simulink library "Driveshaft_ShaftsAll"  (R2026a)
settings: Solver=VariableStepAuto
undefined symbols (not defined in the file): Axle1D, AxleIn, Driveshaft, Housing, Right, Shaft, Shaft1D, Shaft3D, Vehicle, Visual, X, Y, Z
libraries: sm_lib x27, $bdroot x6, fl_lib x4, nesl_utility x2, sm_car_lib x2, Differential_Components x1
Description:
  | Component of Simscape Vehicle Templates Library
  | 
  | Copyright 2018-2026 The MathWorks, Inc.
settings Model: Creator=smiller  LastModifiedBy=smiller

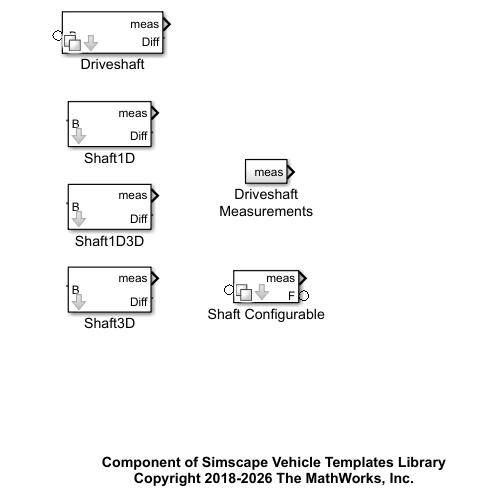
[thumbnail: Simulink's stored preview of the top-level diagram]
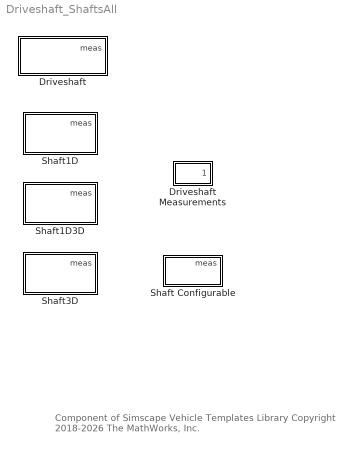
== system Driveshaft_ShaftsAll ==
  note: Component of Simscape Vehicle Templates Library
      | Copyright 2018-2026 The MathWorks, Inc.
  Driveshaft : Subsystem  Variant=on  VariantControl=Variant1  mask(Driveshaft Assembly){popup_leftRight=Right, Driveshaft=Vehicle.Powertrain.Driveline.DriveshaftFR, VariantLabel=Vehicle.Powertrain.Driveline.DriveshaftFR.class.Value, InitTriggerDropdown=1}
      mask prompts: popup_leftRight "Left/Right"; Driveshaft "Driveshaft Parameters"; VariantLabel "Variant Label"; InitTriggerDropdown "Initialization Trigger Dropdown"
      mask help: Models driveshaft and connections to differential and wheels. Joints can be configured to permit plunge at inner or outer joints.
      mask init:
      | curblk = gcb;
      | 
      | % Find other left/right blocks
      | h = sm_car_lib_find_leftright_blocks(curblk);
      | 
      | % Set left/right
      | for i=1:length(h)
      |     try % Avoid setting parameter within library links
      |         set_param(h(i),'popup_leftRight',get_param(curblk,'popup_leftRight'));
      |     end
      | end
      | 
      | % Set variant for this block 
      | set_param(curblk,'LabelModeActiveChoice',VariantLabel);
      | 
      | % Trigger Mask Initialization for 
      | % variant subsystems below this level
      | sm_car_lib_maskInitTrigger(curblk)
      settings: AttributesFormatString=%<ActiveVariant>
      mask TypeOptions popup_leftRight: Left | Right
      mask TypeOptions InitTriggerDropdown: 0 | 1
      mask Display: disp(' ');
  Driveshaft Measurements : Subsystem
  Shaft Configurable : Subsystem  Variant=on  VariantControl=Variant1  mask(Shaft (Configurable)){popup_leftRight=Right, Shaft=Vehicle.Powertrain.Driveline.DriveshaftFL.Shaft, VariantLabel=Vehicle.Powertrain.Driveline.DriveshaftFL.Shaft.class.Value, InitTriggerDropdown=1, clr_shaft=Visual.Driveshaft.clr, opc_shaft=Visual.part.opc, rad_shaft=Visual.Driveshaft.rad}
      mask prompts: popup_leftRight "Left/Right"; Shaft "Shaft Parameters"; VariantLabel "Variant Label"; InitTriggerDropdown "Initialization Trigger Dropdown"; clr_shaft "Color [RGB]"; opc_shaft "Opacity (0-1)"; rad_shaft "Radius (m)"
      mask help: Models a shaft (rigid or flexible).
      mask init:
      | curblk = gcb;
      | 
      | % Find other left/right blocks
      | h = sm_car_lib_find_leftright_blocks(curblk);
      | 
      | % Set left/right
      | for i=1:length(h)
      |     try % Avoid setting parameter within library links
      |         set_param(h(i),'popup_leftRight',get_param(curblk,'popup_leftRight'));
      |     end
      | end
      | 
      | % Set variant for this block 
      | set_param(curblk,'LabelModeActiveChoice',VariantLabel);
      | 
      | % Trigger Mask Initialization for 
      | % variant subsystems below this level
      | sm_car_lib_maskInitTrigger(curblk)
      mask TypeOptions popup_leftRight: Left | Right
      mask TypeOptions InitTriggerDropdown: 0 | 1
      mask DialogControl cont_vis_shaft Prompt: Visualization
      mask Display: disp(' ')
  Shaft1D : Subsystem  VariantControl=Shaft1D  mask(Driveshaft Assembly (1D)){}
      mask help: Models a shaft as a 1D mechanical connection.
  Shaft1D3D : Subsystem  VariantControl=Shaft1D3D  mask(Driveshaft Assembly (1D and 3D)){popup_leftRight=Right, drv_sha_drvsh_m=Driveshaft.Shaft.m.Value, clr_drv_sha_hp=Visual.hp.clr, opc_drv_sha_hp=Visual.hp.opc, rad_drv_sha_hp=Visual.hp.rad, clr_drv_sha_jnt=Visual.DriveshaftCVs.clr, opc_drv_sha_jnt=Visual.part.opc, rad_drv_sha_jnt=Visual.DriveshaftCVs.rad, clr_drv_sha_drvsh=Visual.Driveshaft.clr, opc_drv_sha_drvsh=Visual.part.opc, rad_drv_sha_drvsh=Visual.Driveshaft.rad, len_drv_sha_drvsh=Driveshaft.Shaft.l.Value}
      mask prompts: popup_leftRight "Left/Right"; drv_sha_drvsh_m "Driveshaft Mass (kg)"; len_drv_sha_drvsh "Driveshaft Length (m)"
      mask help: Models a shaft with a 1D mechanical connection for transmitting power and a non-rotating 3D connection for inertia and visualization.
      mask TypeOptions popup_leftRight: AxleInboard/popup_leftRight | Shaft/popup_leftRight | Transaxle/popup_leftRight
      mask TypeOptions drv_sha_drvsh_m: Shaft/shaft_m
      mask TypeOptions clr_drv_sha_hp:
      | Vis HP
      | Transaxle/GraphicDiffuseColor
      mask TypeOptions opc_drv_sha_hp:
      | Vis HP
      | Transaxle/GraphicOpacity
      mask TypeOptions rad_drv_sha_hp:
      | Vis HP
      | Transaxle/SphereRadius
      mask TypeOptions clr_drv_sha_jnt:
      | Vis CV Joint
      | Inboard/GraphicDiffuseColor | Vis CV Joint
      | Outboard/GraphicDiffuseColor
      mask TypeOptions opc_drv_sha_jnt:
      | Vis CV Joint
      | Inboard/GraphicOpacity | Vis CV Joint
      | Outboard/GraphicOpacity
      mask TypeOptions rad_drv_sha_jnt:
      | Vis CV Joint
      | Inboard/SphereRadius | Vis CV Joint
      | Outboard/SphereRadius
      mask TypeOptions clr_drv_sha_drvsh: Shaft/clr_shaft
      mask TypeOptions opc_drv_sha_drvsh: Shaft/opc_shaft
      mask TypeOptions rad_drv_sha_drvsh: Shaft/rad_shaft
      mask TypeOptions len_drv_sha_drvsh: Shaft/len_shaft
      mask DialogControl cont_vis_drv_sha Prompt: Visualization
      mask DialogControl text_vis_drv_sha_clr Prompt: Color [RGB]
      mask DialogControl text_vis_drv_sha_opc Prompt: Opac. (0-1)
      mask DialogControl text_vis_drv_sha_rad Prompt: Radius (m)
      mask DialogControl text_vis_drv_sha_hp Prompt: Hardpoints
      mask DialogControl text_vis_drv_sha_joints Prompt: Joints
      mask DialogControl text_vis_drv_sha_drvsh Prompt: Driveshaft
  Shaft3D : Subsystem  VariantControl=Shaft3D  mask(Driveshaft Assembly (3D)){popup_leftRight=Right, Driveshaft=Driveshaft, InitTriggerDropdown=1, clr_drv_sha_hp=Visual.hp.clr, opc_drv_sha_hp=Visual.hp.opc, rad_drv_sha_hp=Visual.hp.rad, clr_drv_sha_jnt=Visual.DriveshaftCVs.clr, opc_drv_sha_jnt=Visual.part.opc, rad_drv_sha_jnt=Visual.DriveshaftCVs.rad, clr_drv_sha_drvsh=Visual.Driveshaft.clr, opc_drv_sha_drvsh=Visual.part.opc, rad_drv_sha_drvsh=Visual.Driveshaft.rad}
      mask prompts: popup_leftRight "Left/Right"; Driveshaft "Driveshaft Parameters"; InitTriggerDropdown "Initialization Trigger Dropdown"
      mask help: Models a driveshaft assembly with CV joints and a shaft. The joints can be configured to permit plunge at the inboard or outboard joint. The shaft can be rigid or flexible.
      mask init:
      | curblk = gcb;
      | 
      | % Trigger Mask Initialization for 
      | % variant subsystems below this level
      | sm_car_lib_maskInitTrigger(curblk)
      mask TypeOptions popup_leftRight: AxleInboard/popup_leftRight | Shaft/popup_leftRight
      mask TypeOptions InitTriggerDropdown: 0 | 1
      mask TypeOptions clr_drv_sha_hp:
      | Vis HP
      | Transaxle/GraphicDiffuseColor
      mask TypeOptions opc_drv_sha_hp:
      | Vis HP
      | Transaxle/GraphicOpacity
      mask TypeOptions rad_drv_sha_hp:
      | Vis HP
      | Transaxle/SphereRadius
      mask TypeOptions clr_drv_sha_jnt:
      | Vis CV Joint
      | Inboard/GraphicDiffuseColor | Vis CV Joint
      | Outboard/GraphicDiffuseColor
      mask TypeOptions opc_drv_sha_jnt:
      | Vis CV Joint
      | Inboard/GraphicOpacity | Vis CV Joint
      | Outboard/GraphicOpacity
      mask TypeOptions rad_drv_sha_jnt:
      | Vis CV Joint
      | Inboard/SphereRadius | Vis CV Joint
      | Outboard/SphereRadius
      mask TypeOptions clr_drv_sha_drvsh: Shaft/clr_shaft
      mask TypeOptions opc_drv_sha_drvsh: Shaft/opc_shaft
      mask TypeOptions rad_drv_sha_drvsh: Shaft/rad_shaft
      mask DialogControl cont_vis_drv_sha Prompt: Visualization
      mask DialogControl text_vis_drv_sha_clr Prompt: Color [RGB]
      mask DialogControl text_vis_drv_sha_opc Prompt: Opac. (0-1)
      mask DialogControl text_vis_drv_sha_rad Prompt: Radius (m)
      mask DialogControl text_vis_drv_sha_hp Prompt: Hardpoints
      mask DialogControl text_vis_drv_sha_joints Prompt: Joints
      mask DialogControl text_vis_drv_sha_drvsh Prompt: Driveshaft

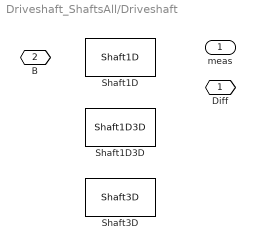
== system Driveshaft_ShaftsAll/Driveshaft ==
  Shaft1D : $bdroot/Shaft1D  VariantControl=Shaft1D
  Shaft1D3D : $bdroot/Shaft1D3D  VariantControl=Shaft1D3D  popup_leftRight=Right  drv_sha_drvsh_m=Driveshaft.Shaft.m.Value  clr_drv_sha_hp=Visual.hp.clr  opc_drv_sha_hp=Visual.hp.opc  rad_drv_sha_hp=Visual.hp.rad  clr_drv_sha_jnt=Visual.DriveshaftCVs.clr  opc_drv_sha_jnt=Visual.part.opc  rad_drv_sha_jnt=Visual.DriveshaftCVs.rad  clr_drv_sha_drvsh=Visual.Driveshaft.clr  opc_drv_sha_drvsh=Visual.part.opc  rad_drv_sha_drvsh=Visual.Driveshaft.rad  len_drv_sha_drvsh=Driveshaft.Shaft.l.Value
  Shaft3D : $bdroot/Shaft3D  VariantControl=Shaft3D  popup_leftRight=Right  Driveshaft=Driveshaft  InitTriggerDropdown=1  clr_drv_sha_hp=Visual.hp.clr  opc_drv_sha_hp=Visual.hp.opc  rad_drv_sha_hp=Visual.hp.rad  clr_drv_sha_jnt=Visual.DriveshaftCVs.clr  opc_drv_sha_jnt=Visual.part.opc  rad_drv_sha_jnt=Visual.DriveshaftCVs.rad  clr_drv_sha_drvsh=Visual.Driveshaft.clr  opc_drv_sha_drvsh=Visual.part.opc  rad_drv_sha_drvsh=Visual.Driveshaft.rad
  Diff : PMIOPort  Side=Right
  " B" : PMIOPort  Port=2  Side=Left
  meas : Outport  VectorParamsAs1DForOutWhenUnconnected=off

== system Driveshaft_ShaftsAll/Driveshaft Measurements ==
  Bus Creator : BusCreator  Inputs=2
  Zero : Constant  Value=0  OutDataTypeStr=Inherit: Inherit via back propagation
  Zero1 : Constant  Value=0  OutDataTypeStr=Inherit: Inherit via back propagation
  meas : Outport  VectorParamsAs1DForOutWhenUnconnected=off
  wires:
  Bus Creator/1 -> meas/1
  Zero1/1 -> Bus Creator/2  "q"
  Zero/1 -> Bus Creator/1  "w"

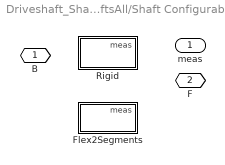
== system Driveshaft_ShaftsAll/Shaft Configurable ==
  Flex2Segments : Subsystem  VariantControl=Flex2Segments  mask{popup_leftRight=Right, shaft_m=Shaft.m.Value, len_shaft=Shaft.l.Value, shaft_K=Shaft.K.Value, shaft_d=Shaft.d.Value, clr_shaft=clr_shaft, opc_shaft=opc_shaft, rad_shaft=rad_shaft}
      mask prompts: popup_leftRight "Left/Right"; shaft_m "Shaft Mass (kg)"; len_shaft "Shaft Length (m)"; shaft_K "Shaft Stiffness (N*m/rad)"; shaft_d "Shaft Damping (N*m/(rad/s))"; clr_shaft "Color [RGB]"; opc_shaft "Opacity (0-1)"; rad_shaft "Radius (m)"
      mask init:
      | if(popup_leftRight == 1)
      |     rhs_shaft = 1;
      | elseif(popup_leftRight == 2)
      |     rhs_shaft = -1;
      | end
      mask TypeOptions popup_leftRight: Left | Right
      mask TypeOptions shaft_m: Shaft/Mass
      mask TypeOptions shaft_K:
      | Revolute
      | Flex/SpringStiffness
      mask TypeOptions shaft_d:
      | Revolute
      | Flex/DampingCoefficient
      mask TypeOptions clr_shaft: Shaft/GraphicDiffuseColor
      mask TypeOptions opc_shaft: Shaft/GraphicOpacity
      mask TypeOptions rad_shaft: Shaft/CylinderRadius
      mask DialogControl cont_vis_shaft Prompt: Visualization
  Rigid : Subsystem  VariantControl=Rigid  mask{popup_leftRight=Right, shaft_m=Shaft.m.Value, len_shaft=Shaft.l.Value, clr_shaft=clr_shaft, opc_shaft=opc_shaft, rad_shaft=rad_shaft}
      mask prompts: popup_leftRight "Left/Right"; shaft_m "Shaft Mass (kg)"; len_shaft "Shaft Length (m)"; clr_shaft "Color [RGB]"; opc_shaft "Opacity (0-1)"; rad_shaft "Radius (m)"
      mask init:
      | if(popup_leftRight == 1)
      |     rhs_shaft = 1;
      | elseif(popup_leftRight == 2)
      |     rhs_shaft = -1;
      | end
      mask TypeOptions popup_leftRight: Left | Right
      mask TypeOptions shaft_m: Shaft/Mass
      mask TypeOptions clr_shaft: Shaft/GraphicDiffuseColor
      mask TypeOptions opc_shaft: Shaft/GraphicOpacity
      mask TypeOptions rad_shaft: Shaft/CylinderRadius
      mask DialogControl cont_vis_shaft Prompt: Visualization
  " B" : PMIOPort  Side=Left
  " F" : PMIOPort  Port=2  Side=Right
  " meas" : Outport  VectorParamsAs1DForOutWhenUnconnected=off

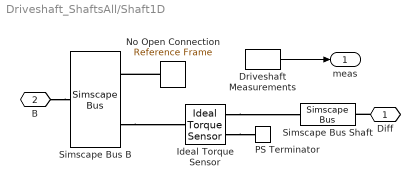
== system Driveshaft_ShaftsAll/Shaft1D ==
  Driveshaft Measurements : $bdroot/Driveshaft Measurements  SystemSampleTime=-1  VariantActivationTime=update diagram  EmptyChoice=off  PassThrough=off  PassThroughVariantControl=(default)  EmptyChoiceVariantControl=(default)  AllowFlexibleInterface=on  Latency=0  AutoFrameSizeCalculation=off
  Ideal Torque Sensor : fl_lib/Mechanical/Mechanical Sensors/Ideal Torque Sensor
  No Open Connection : sm_lib/Frames and Transforms/Reference Frame
  PS Terminator : fl_lib/Physical Signals/Sinks/PS Terminator
  Simscape Bus B : SimscapeBus  HierarchyStrings=AxleIn;Axle1D
  Simscape Bus Shaft : SimscapeBus  HierarchyStrings=Shaft1D
  Diff : PMIOPort  Side=Right
  B : PMIOPort  Port=2  Side=Left
  meas : Outport  VectorParamsAs1DForOutWhenUnconnected=off
  wires:
  Driveshaft Measurements/1 -> meas/1
  connections:
  No Open Connection/RConn1 -- Simscape Bus B/LConn1
  B/RConn1 -- Simscape Bus B/RConn1
  Ideal Torque Sensor/RConn2 -- PS Terminator/LConn1
  Diff/RConn1 -- Simscape Bus Shaft/RConn1
  Ideal Torque Sensor/RConn1 -- Simscape Bus Shaft/LConn1
  Simscape Bus B/LConn2 -- Ideal Torque Sensor/LConn1

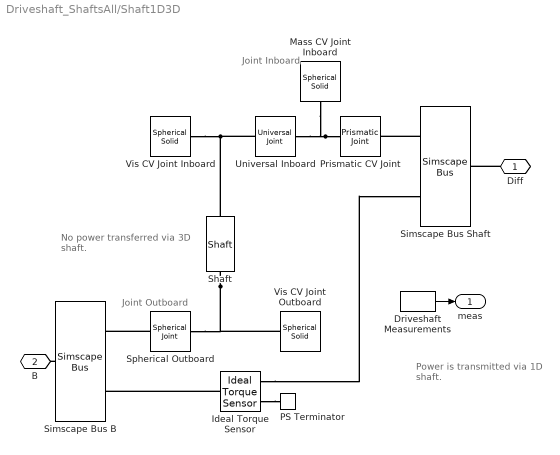
== system Driveshaft_ShaftsAll/Shaft1D3D ==
  note: Joint Inboard
  note: Joint Outboard
  note: No power transferred
      | via 3D shaft.
  note: Power is transmitted via 1D shaft.
  Driveshaft Measurements : $bdroot/Driveshaft Measurements  SystemSampleTime=-1  VariantActivationTime=update diagram  EmptyChoice=off  PassThrough=off  PassThroughVariantControl=(default)  EmptyChoiceVariantControl=(default)  AllowFlexibleInterface=on  Latency=0  AutoFrameSizeCalculation=off
  Ideal Torque Sensor : fl_lib/Mechanical/Mechanical Sensors/Ideal Torque Sensor
  Mass CV Joint Inboard : sm_lib/Body Elements/Spherical Solid  SphereRadius=5e-3  SphereRadiusUnits=m  ExportEntireGeometry=off  InertiaType=CalculateFromGeometry  BasedOnType=Density  Density=1000  DensityUnits=kg/m^3  Mass=1  MassUnits=kg  CenterOfMass=[0 0 0]  CenterOfMassUnits=m  MomentsOfInertia=[1 1 1]  MomentsOfInertiaUnits=kg*m^2  ProductsOfInertia=[0 0 0]  ProductsOfInertiaUnits=kg*m^2  GraphicType=FromGeometry  MarkerShape=Sphere  MarkerSize=10  GraphicVisPropType=SimpleVisualProperties  GraphicDiffuseColor=[0.5 0.5 0.5]  GraphicOpacity=1  GraphicSpecularColor=[0.5 0.5 0.5 1.0]  GraphicAmbientColor=[0.15 0.15 0.15 1.0]  GraphicEmissiveColor=[0.0 0.0 0.0 1.0]  GraphicShininess=75  DoExposeReferenceFrame=on  SerializedFrames=<Frames/>
  PS Terminator : fl_lib/Physical Signals/Sinks/PS Terminator
  Prismatic CV Joint : sm_lib/Joints/Prismatic Joint  JointMode=Normal  CompositeWrenchDir=FollowerOnBase  CompositeWrenchFrame=BaseFrame  SenseConstraintForce=off  SenseConstraintTorque=off  SenseTotalForce=off  SenseTotalTorque=off  PositionTargetSpecify=off  PositionTargetPriority=High  PositionTargetValue=0  PositionTargetValueUnits=m  VelocityTargetSpecify=off  VelocityTargetPriority=High  VelocityTargetValue=0  VelocityTargetValueUnits=m/s  EquilibriumPosition=0  EquilibriumPositionUnits=m  SpringStiffness=0  SpringStiffnessUnits=N/m  DampingCoefficient=0  DampingCoefficientUnits=N/(m/s)  LowerLimitSpecify=off  LowerLimitBound=-1  LowerLimitBoundUnits=m  LowerLimitStiffness=1e6  LowerLimitStiffnessUnits=N/m  LowerLimitDamping=1e3  LowerLimitDampingUnits=N/(m/s)  LowerLimitTransitionRegionWidth=1e-4  LowerLimitTransitionRegionWidthUnits=m  UpperLimitSpecify=off  UpperLimitBound=1  UpperLimitBoundUnits=m  UpperLimitStiffness=1e6  UpperLimitStiffnessUnits=N/m  UpperLimitDamping=1e3  UpperLimitDampingUnits=N/(m/s)  UpperLimitTransitionRegionWidth=1e-4  UpperLimitTransitionRegionWidthUnits=m  TorqueActuationMode=NoTorque  MotionActuationMode=ComputedMotion  SensePosition=off  SenseVelocity=off  SenseAcceleration=off  SenseTorqueForce=off  SenseLowerLimitTorqueForce=off  SenseUpperLimitTorqueForce=off
  Shaft : Differential_Components/Shaft  popup_leftRight=Right  shaft_m=drv_sha_drvsh_m  len_shaft=len_drv_sha_drvsh  clr_shaft=clr_drv_sha_drvsh  opc_shaft=opc_drv_sha_drvsh  rad_shaft=rad_drv_sha_drvsh
  Simscape Bus B : SimscapeBus  HierarchyStrings=AxleIn;Axle1D
  Simscape Bus Shaft : SimscapeBus  HierarchyStrings=Shaft3D;Shaft1D
  Spherical Outboard : sm_lib/Joints/Spherical Joint  JointMode=Normal  CompositeWrenchDir=FollowerOnBase  CompositeWrenchFrame=BaseFrame  SenseConstraintForce=off  SenseConstraintTorque=off  SenseTotalForce=off  SenseTotalTorque=off  PositionTargetSpecify=off  PositionTargetPriority=High  PositionTargetRotationMethod=None  PositionTargetFollAlignAxisA=+X  PositionTargetBaseAlignAxisA=+Y  PositionTargetFollAlignAxisB=+Y  PositionTargetBaseAlignAxisB=+Z  PositionTargetRotationStandardAxis=+Z  PositionTargetRotationAngle=0.0  PositionTargetRotationAngleUnits=deg  PositionTargetRotationArbitraryAxis=[0 0 1]  PositionTargetRotationSequenceAxes=FollowerAxes  PositionTargetRotationSequence=XYX  PositionTargetRotationSequenceAngles=[0 0 0]  PositionTargetRotationSequenceAnglesUnits=deg  PositionTargetRotationMatrix=[1 0 0; 0 1 0; 0 0 1]  PositionTargetQuaternion=[1 0 0 0]  VelocityTargetSpecify=off  VelocityTargetPriority=High  VelocityTargetValue=[0 0 0]  VelocityTargetValueUnits=deg/s  VelocityTargetInFollowerFrame=on  EqPosRotationMethod=None  EqPosFollAlignAxisA=+X  EqPosBaseAlignAxisA=+Y  EqPosFollAlignAxisB=+Y  EqPosBaseAlignAxisB=+Z  EqPosRotationStandardAxis=+Z  EqPosRotationAngle=0.0  EqPosRotationAngleUnits=deg  EqPosRotationArbitraryAxis=[0 0 1]  EqPosRotationSequenceAxes=FollowerAxes  EqPosRotationSequence=XYX  EqPosRotationSequenceAngles=[0 0 0]  EqPosRotationSequenceAnglesUnits=deg  EqPosRotationMatrix=[1 0 0; 0 1 0; 0 0 1]  EqPosQuaternion=[1 0 0 0]  SpringStiffness=0  SpringStiffnessUnits=N*m/deg  DampingCoefficient=0  DampingCoefficientUnits=N*m/(deg/s)  LowerLimitSpecify=off  LowerLimitBound=15  LowerLimitBoundUnits=deg  LowerLimitStiffness=1e4  LowerLimitStiffnessUnits=N*m/deg  LowerLimitDamping=10  LowerLimitDampingUnits=N*m/(deg/s)  LowerLimitTransitionRegionWidth=0.1  LowerLimitTransitionRegionWidthUnits=deg  UpperLimitSpecify=off  UpperLimitBound=45  UpperLimitBoundUnits=deg  UpperLimitStiffness=1e4  UpperLimitStiffnessUnits=N*m/deg  UpperLimitDamping=10  UpperLimitDampingUnits=N*m/(deg/s)  UpperLimitTransitionRegionWidth=0.1  UpperLimitTransitionRegionWidthUnits=deg  TorqueActuationMode=NoTorque  ActuateTorqueX=off  ActuateTorqueY=off  ActuateTorqueZ=off  ActuateTorque=off  ActuationFrame=BaseFrame  SensePosition=off  SenseVelocityX=off  SenseVelocityY=off  SenseVelocityZ=off  SenseVelocity=off  SenseAccelerationX=off  SenseAccelerationY=off  SenseAccelerationZ=off  SenseAcceleration=off  SenseLowerLimitTorqueMag=off  SenseUpperLimitTorqueMag=off  SensingFrame=BaseFrame
  Universal Inboard : sm_lib/Joints/Universal Joint  JointMode=Normal  CompositeWrenchDir=FollowerOnBase  CompositeWrenchFrame=BaseFrame  SenseConstraintForce=off  SenseConstraintTorque=off  SenseTotalForce=off  SenseTotalTorque=off  RxPositionTargetSpecify=off  RxPositionTargetPriority=High  RxPositionTargetValue=0  RxPositionTargetValueUnits=deg  RxVelocityTargetSpecify=off  RxVelocityTargetPriority=High  RxVelocityTargetValue=0  RxVelocityTargetValueUnits=deg/s  RxEquilibriumPosition=0  RxEquilibriumPositionUnits=deg  RxSpringStiffness=0  RxSpringStiffnessUnits=N*m/deg  RxDampingCoefficient=0  RxDampingCoefficientUnits=N*m/(deg/s)  RxLowerLimitSpecify=off  RxLowerLimitBound=-90  RxLowerLimitBoundUnits=deg  RxLowerLimitStiffness=1e4  RxLowerLimitStiffnessUnits=N*m/deg  RxLowerLimitDamping=10  RxLowerLimitDampingUnits=N*m/(deg/s)  RxLowerLimitTransitionRegionWidth=0.1  RxLowerLimitTransitionRegionWidthUnits=deg  RxUpperLimitSpecify=off  RxUpperLimitBound=90  RxUpperLimitBoundUnits=deg  RxUpperLimitStiffness=1e4  RxUpperLimitStiffnessUnits=N*m/deg  RxUpperLimitDamping=10  RxUpperLimitDampingUnits=N*m/(deg/s)  RxUpperLimitTransitionRegionWidth=0.1  RxUpperLimitTransitionRegionWidthUnits=deg  RxTorqueActuationMode=NoTorque  RxMotionActuationMode=ComputedMotion  RxSensePosition=off  RxSenseVelocity=off  RxSenseAcceleration=off  RxSenseTorqueForce=off  RxSenseLowerLimitTorqueForce=off  RxSenseUpperLimitTorqueForce=off  RyPositionTargetSpecify=off  RyPositionTargetPriority=High  RyPositionTargetValue=0  RyPositionTargetValueUnits=deg  RyVelocityTargetSpecify=off  RyVelocityTargetPriority=High  RyVelocityTargetValue=0  RyVelocityTargetValueUnits=deg/s  RyEquilibriumPosition=0  RyEquilibriumPositionUnits=deg  RySpringStiffness=0  RySpringStiffnessUnits=N*m/deg  RyDampingCoefficient=0  RyDampingCoefficientUnits=N*m/(deg/s)  RyLowerLimitSpecify=off  RyLowerLimitBound=-90  RyLowerLimitBoundUnits=deg  RyLowerLimitStiffness=1e4  RyLowerLimitStiffnessUnits=N*m/deg  RyLowerLimitDamping=10  RyLowerLimitDampingUnits=N*m/(deg/s)  RyLowerLimitTransitionRegionWidth=0.1  RyLowerLimitTransitionRegionWidthUnits=deg  RyUpperLimitSpecify=off  RyUpperLimitBound=90  RyUpperLimitBoundUnits=deg  RyUpperLimitStiffness=1e4  RyUpperLimitStiffnessUnits=N*m/deg  RyUpperLimitDamping=10  RyUpperLimitDampingUnits=N*m/(deg/s)  RyUpperLimitTransitionRegionWidth=0.1  RyUpperLimitTransitionRegionWidthUnits=deg  RyTorqueActuationMode=NoTorque  RyMotionActuationMode=ComputedMotion  RySensePosition=off  RySenseVelocity=off  RySenseAcceleration=off  RySenseTorqueForce=off  RySenseLowerLimitTorqueForce=off  RySenseUpperLimitTorqueForce=off
  Vis CV Joint Inboard : sm_lib/Body Elements/Spherical Solid  SphereRadius=rad_drv_sha_jnt  SphereRadiusUnits=m  ExportEntireGeometry=off  InertiaType=CalculateFromGeometry  BasedOnType=Density  Density=0  DensityUnits=kg/m^3  Mass=1  MassUnits=kg  CenterOfMass=[0 0 0]  CenterOfMassUnits=m  MomentsOfInertia=[1 1 1]  MomentsOfInertiaUnits=kg*m^2  ProductsOfInertia=[0 0 0]  ProductsOfInertiaUnits=kg*m^2  GraphicType=FromGeometry  MarkerShape=Sphere  MarkerSize=10  GraphicVisPropType=SimpleVisualProperties  GraphicDiffuseColor=clr_drv_sha_jnt  GraphicOpacity=opc_drv_sha_jnt  GraphicSpecularColor=[0.5 0.5 0.5 1.0]  GraphicAmbientColor=[0.15 0.15 0.15 1.0]  GraphicEmissiveColor=[0.0 0.0 0.0 1.0]  GraphicShininess=75  DoExposeReferenceFrame=on  SerializedFrames=<Frames/>
  Vis CV Joint Outboard : sm_lib/Body Elements/Spherical Solid  SphereRadius=rad_drv_sha_jnt  SphereRadiusUnits=m  ExportEntireGeometry=off  InertiaType=CalculateFromGeometry  BasedOnType=Density  Density=0  DensityUnits=kg/m^3  Mass=1  MassUnits=kg  CenterOfMass=[0 0 0]  CenterOfMassUnits=m  MomentsOfInertia=[1 1 1]  MomentsOfInertiaUnits=kg*m^2  ProductsOfInertia=[0 0 0]  ProductsOfInertiaUnits=kg*m^2  GraphicType=FromGeometry  MarkerShape=Sphere  MarkerSize=10  GraphicVisPropType=SimpleVisualProperties  GraphicDiffuseColor=clr_drv_sha_jnt  GraphicOpacity=opc_drv_sha_jnt  GraphicSpecularColor=[0.5 0.5 0.5 1.0]  GraphicAmbientColor=[0.15 0.15 0.15 1.0]  GraphicEmissiveColor=[0.0 0.0 0.0 1.0]  GraphicShininess=75  DoExposeReferenceFrame=on  SerializedFrames=<Frames/>
  Diff : PMIOPort  Side=Right
  B : PMIOPort  Port=2  Side=Left
  meas : Outport  VectorParamsAs1DForOutWhenUnconnected=off
  wires:
  Driveshaft Measurements/1 -> meas/1
  connections:
  Ideal Torque Sensor/RConn2 -- PS Terminator/LConn1
  Ideal Torque Sensor/RConn1 -- Simscape Bus Shaft/LConn2
  Diff/RConn1 -- Simscape Bus Shaft/RConn1
  Ideal Torque Sensor/LConn1 -- Simscape Bus B/LConn2
  Simscape Bus B/RConn1 -- B/RConn1
  Vis CV Joint Inboard/RConn1 -- Universal Inboard/LConn1 -- Shaft/RConn1
  Prismatic CV Joint/LConn1 -- Universal Inboard/RConn1 -- Mass CV Joint Inboard/RConn1
  Spherical Outboard/LConn1 -- Simscape Bus B/LConn1
  Shaft/LConn1 -- Vis CV Joint Outboard/RConn1 -- Spherical Outboard/RConn1
  Simscape Bus Shaft/LConn1 -- Prismatic CV Joint/RConn1

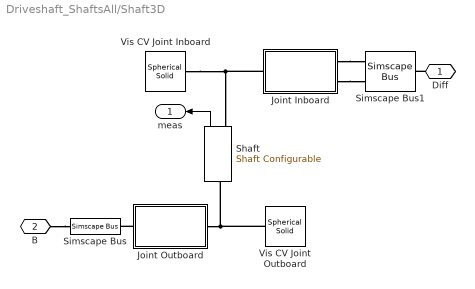
== system Driveshaft_ShaftsAll/Shaft3D ==
  Joint Inboard : Subsystem  Variant=on  VariantControl=Variant1  mask{VariantLabel=Driveshaft.JointInboard.class.Value, InitTriggerDropdown=1}
      mask prompts: VariantLabel "Variant Label"; InitTriggerDropdown "Initialization Trigger Dropdown"
      mask init:
      | curblk = gcb;
      | 
      | % Set variant for this block 
      | set_param(curblk,'LabelModeActiveChoice',VariantLabel);
      | 
      | % Trigger Mask Initialization for 
      | % variant subsystems below this level
      | sm_car_lib_maskInitTrigger(curblk)
      settings: AttributesFormatString=%<ActiveVariant>
      mask TypeOptions InitTriggerDropdown: 0 | 1
      mask Display: disp(' ');
  Joint Outboard : Subsystem  Variant=on  VariantControl=Variant1  mask{VariantLabel=Driveshaft.JointOutboard.class.Value, InitTriggerDropdown=1}
      mask prompts: VariantLabel "Variant Label"; InitTriggerDropdown "Initialization Trigger Dropdown"
      mask init: same as Driveshaft_ShaftsAll/Shaft3D/Joint Inboard
      settings: AttributesFormatString=%<ActiveVariant>
      mask TypeOptions InitTriggerDropdown: 0 | 1
      mask Display: disp(' ');
  Shaft : $bdroot/Shaft Configurable  VariantControl=Variant1  popup_leftRight=Right  Shaft=Driveshaft.Shaft  VariantLabel=Driveshaft.Shaft.class.Value  InitTriggerDropdown=1  clr_shaft=clr_drv_sha_drvsh  opc_shaft=opc_drv_sha_drvsh  rad_shaft=rad_drv_sha_drvsh
      settings: AttributesFormatString=%<ActiveVariant>
  Simscape Bus : SimscapeBus  HierarchyStrings=AxleIn
  Simscape Bus1 : SimscapeBus  HierarchyStrings=Shaft;Housing
  Vis CV Joint Inboard : sm_lib/Body Elements/Spherical Solid  SphereRadius=rad_drv_sha_jnt  SphereRadiusUnits=m  ExportEntireGeometry=off  InertiaType=CalculateFromGeometry  BasedOnType=Density  Density=0  DensityUnits=kg/m^3  Mass=1  MassUnits=kg  CenterOfMass=[0 0 0]  CenterOfMassUnits=m  MomentsOfInertia=[1 1 1]  MomentsOfInertiaUnits=kg*m^2  ProductsOfInertia=[0 0 0]  ProductsOfInertiaUnits=kg*m^2  GraphicType=FromGeometry  MarkerShape=Sphere  MarkerSize=10  GraphicVisPropType=SimpleVisualProperties  GraphicDiffuseColor=clr_drv_sha_jnt  GraphicOpacity=opc_drv_sha_jnt  GraphicSpecularColor=[0.5 0.5 0.5 1.0]  GraphicAmbientColor=[0.15 0.15 0.15 1.0]  GraphicEmissiveColor=[0.0 0.0 0.0 1.0]  GraphicShininess=75  DoExposeReferenceFrame=on  SerializedFrames=<Frames/>
  Vis CV Joint Outboard : sm_lib/Body Elements/Spherical Solid  SphereRadius=rad_drv_sha_jnt  SphereRadiusUnits=m  ExportEntireGeometry=off  InertiaType=CalculateFromGeometry  BasedOnType=Density  Density=0  DensityUnits=kg/m^3  Mass=1  MassUnits=kg  CenterOfMass=[0 0 0]  CenterOfMassUnits=m  MomentsOfInertia=[1 1 1]  MomentsOfInertiaUnits=kg*m^2  ProductsOfInertia=[0 0 0]  ProductsOfInertiaUnits=kg*m^2  GraphicType=FromGeometry  MarkerShape=Sphere  MarkerSize=10  GraphicVisPropType=SimpleVisualProperties  GraphicDiffuseColor=clr_drv_sha_jnt  GraphicOpacity=opc_drv_sha_jnt  GraphicSpecularColor=[0.5 0.5 0.5 1.0]  GraphicAmbientColor=[0.15 0.15 0.15 1.0]  GraphicEmissiveColor=[0.0 0.0 0.0 1.0]  GraphicShininess=75  DoExposeReferenceFrame=on  SerializedFrames=<Frames/>
  Diff : PMIOPort  Side=Right
  B : PMIOPort  Port=2  Side=Left
  meas : Outport  VectorParamsAs1DForOutWhenUnconnected=off
  wires:
  Shaft/1 -> meas/1
  connections:
  Joint Outboard/LConn1 -- Simscape Bus/LConn1
  Joint Outboard/RConn1 -- Shaft/LConn1 -- Vis CV Joint Outboard/RConn1
  Joint Inboard/RConn2 -- Simscape Bus1/LConn2
  Joint Inboard/RConn1 -- Simscape Bus1/LConn1
  Joint Inboard/LConn1 -- Shaft/RConn1 -- Vis CV Joint Inboard/RConn1
  Diff/RConn1 -- Simscape Bus1/RConn1
  B/RConn1 -- Simscape Bus/RConn1

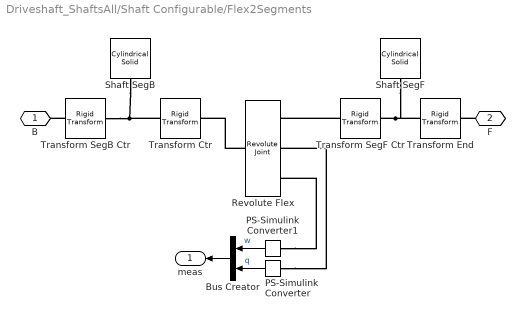
== system Driveshaft_ShaftsAll/Shaft Configurable/Flex2Segments ==
  Bus Creator : BusCreator  Inputs=2
  PS-Simulink Converter : nesl_utility/PS-Simulink Converter  PhysicalDomain=network_engine_domain  SubClassName=ps_output  LeftPortType=input  RightPortType=output  PseudoPeriodic=off  Frequencies=[]  VectorFormat=1-D array  Unit=rad  AffineConversion=off
  PS-Simulink Converter1 : nesl_utility/PS-Simulink Converter  PhysicalDomain=network_engine_domain  SubClassName=ps_output  LeftPortType=input  RightPortType=output  PseudoPeriodic=off  Frequencies=[]  VectorFormat=1-D array  Unit=rad/s  AffineConversion=off
  Revolute Flex : sm_lib/Joints/Revolute Joint  JointMode=Normal  CompositeWrenchDir=FollowerOnBase  CompositeWrenchFrame=BaseFrame  SenseConstraintForce=off  SenseConstraintTorque=off  SenseTotalForce=off  SenseTotalTorque=off  PositionTargetSpecify=off  PositionTargetPriority=High  PositionTargetValue=0  PositionTargetValueUnits=deg  VelocityTargetSpecify=off  VelocityTargetPriority=High  VelocityTargetValue=0  VelocityTargetValueUnits=deg/s  EquilibriumPosition=0  EquilibriumPositionUnits=deg  SpringStiffness=shaft_K  SpringStiffnessUnits=N*m/rad  DampingCoefficient=shaft_d  DampingCoefficientUnits=N*m/(rad/s)  LowerLimitSpecify=off  LowerLimitBound=-90  LowerLimitBoundUnits=deg  LowerLimitStiffness=1e4  LowerLimitStiffnessUnits=N*m/deg  LowerLimitDamping=10  LowerLimitDampingUnits=N*m/(deg/s)  LowerLimitTransitionRegionWidth=0.1  LowerLimitTransitionRegionWidthUnits=deg  UpperLimitSpecify=off  UpperLimitBound=90  UpperLimitBoundUnits=deg  UpperLimitStiffness=1e4  UpperLimitStiffnessUnits=N*m/deg  UpperLimitDamping=10  UpperLimitDampingUnits=N*m/(deg/s)  UpperLimitTransitionRegionWidth=0.1  UpperLimitTransitionRegionWidthUnits=deg  TorqueActuationMode=NoTorque  MotionActuationMode=ComputedMotion  SensePosition=on  SenseVelocity=on  SenseAcceleration=off  SenseTorqueForce=off  SenseLowerLimitTorqueForce=off  SenseUpperLimitTorqueForce=off
  Shaft SegB : sm_lib/Body Elements/Cylindrical Solid  CylinderRadius=rad_shaft  CylinderRadiusUnits=m  CylinderLength=len_shaft/2  CylinderLengthUnits=m  ExportEntireGeometry=off  InertiaType=CalculateFromGeometry  BasedOnType=Mass  Density=1000  DensityUnits=kg/m^3  Mass=shaft_m  MassUnits=kg  CenterOfMass=[0 0 0]  CenterOfMassUnits=m  MomentsOfInertia=[1 1 1]  MomentsOfInertiaUnits=kg*m^2  ProductsOfInertia=[0 0 0]  ProductsOfInertiaUnits=kg*m^2  GraphicType=FromGeometry  MarkerShape=Sphere  MarkerSize=10  GraphicVisPropType=SimpleVisualProperties  GraphicDiffuseColor=clr_shaft  GraphicOpacity=opc_shaft  GraphicSpecularColor=[0.5 0.5 0.5 1.0]  GraphicAmbientColor=[0.15 0.15 0.15 1.0]  GraphicEmissiveColor=[0.0 0.0 0.0 1.0]  GraphicShininess=75  DoExposeReferenceFrame=on  SerializedFrames=<Frames/>
  Shaft SegF : sm_lib/Body Elements/Cylindrical Solid  CylinderRadius=rad_shaft  CylinderRadiusUnits=m  CylinderLength=len_shaft/2  CylinderLengthUnits=m  ExportEntireGeometry=off  InertiaType=CalculateFromGeometry  BasedOnType=Mass  Density=1000  DensityUnits=kg/m^3  Mass=shaft_m  MassUnits=kg  CenterOfMass=[0 0 0]  CenterOfMassUnits=m  MomentsOfInertia=[1 1 1]  MomentsOfInertiaUnits=kg*m^2  ProductsOfInertia=[0 0 0]  ProductsOfInertiaUnits=kg*m^2  GraphicType=FromGeometry  MarkerShape=Sphere  MarkerSize=10  GraphicVisPropType=SimpleVisualProperties  GraphicDiffuseColor=clr_shaft  GraphicOpacity=opc_shaft  GraphicSpecularColor=[0.5 0.5 0.5 1.0]  GraphicAmbientColor=[0.15 0.15 0.15 1.0]  GraphicEmissiveColor=[0.0 0.0 0.0 1.0]  GraphicShininess=75  DoExposeReferenceFrame=on  SerializedFrames=<Frames/>
  Transform Ctr : sm_lib/Frames and Transforms/Rigid Transform  RotationMethod=None  FollAlignAxisA=+X  BaseAlignAxisA=+Y  FollAlignAxisB=+Y  BaseAlignAxisB=+Z  RotationStandardAxis=+Y  RotationAngle=0  RotationAngleUnits=deg  RotationArbitraryAxis=[0 0 1]  RotationSequenceAxes=FollowerAxes  RotationSequence=XYX  RotationSequenceAngles=[0 0 0]  RotationSequenceAnglesUnits=deg  RotationMatrix=[1 0 0; 0 1 0; 0 0 1]  Quaternion=[1 0 0 0]  TranslationMethod=StandardAxis  TranslationCartesianOffset=[0 0 0]  TranslationCartesianOffsetUnits=m  TranslationStandardAxis=-Z  TranslationStandardOffset=len_shaft/4*rhs_shaft  TranslationStandardOffsetUnits=m  TranslationROffset=0  TranslationROffsetUnits=m  TranslationThetaOffset=0  TranslationThetaOffsetUnits=deg  TranslationZOffset=0  TranslationZOffsetUnits=m
  Transform End : sm_lib/Frames and Transforms/Rigid Transform  RotationMethod=None  FollAlignAxisA=+X  BaseAlignAxisA=+Y  FollAlignAxisB=+Y  BaseAlignAxisB=+Z  RotationStandardAxis=+Y  RotationAngle=0  RotationAngleUnits=deg  RotationArbitraryAxis=[0 0 1]  RotationSequenceAxes=FollowerAxes  RotationSequence=XYX  RotationSequenceAngles=[0 0 0]  RotationSequenceAnglesUnits=deg  RotationMatrix=[1 0 0; 0 1 0; 0 0 1]  Quaternion=[1 0 0 0]  TranslationMethod=StandardAxis  TranslationCartesianOffset=[0 0 0]  TranslationCartesianOffsetUnits=m  TranslationStandardAxis=-Z  TranslationStandardOffset=len_shaft/4*rhs_shaft  TranslationStandardOffsetUnits=m  TranslationROffset=0  TranslationROffsetUnits=m  TranslationThetaOffset=0  TranslationThetaOffsetUnits=deg  TranslationZOffset=0  TranslationZOffsetUnits=m
  Transform SegB Ctr : sm_lib/Frames and Transforms/Rigid Transform  RotationMethod=None  FollAlignAxisA=+X  BaseAlignAxisA=+Y  FollAlignAxisB=+Y  BaseAlignAxisB=+Z  RotationStandardAxis=+Y  RotationAngle=0  RotationAngleUnits=deg  RotationArbitraryAxis=[0 0 1]  RotationSequenceAxes=FollowerAxes  RotationSequence=XYX  RotationSequenceAngles=[0 0 0]  RotationSequenceAnglesUnits=deg  RotationMatrix=[1 0 0; 0 1 0; 0 0 1]  Quaternion=[1 0 0 0]  TranslationMethod=StandardAxis  TranslationCartesianOffset=[0 0 0]  TranslationCartesianOffsetUnits=m  TranslationStandardAxis=-Z  TranslationStandardOffset=len_shaft/4*rhs_shaft  TranslationStandardOffsetUnits=m  TranslationROffset=0  TranslationROffsetUnits=m  TranslationThetaOffset=0  TranslationThetaOffsetUnits=deg  TranslationZOffset=0  TranslationZOffsetUnits=m
  Transform SegF Ctr : sm_lib/Frames and Transforms/Rigid Transform  RotationMethod=None  FollAlignAxisA=+X  BaseAlignAxisA=+Y  FollAlignAxisB=+Y  BaseAlignAxisB=+Z  RotationStandardAxis=+Y  RotationAngle=0  RotationAngleUnits=deg  RotationArbitraryAxis=[0 0 1]  RotationSequenceAxes=FollowerAxes  RotationSequence=XYX  RotationSequenceAngles=[0 0 0]  RotationSequenceAnglesUnits=deg  RotationMatrix=[1 0 0; 0 1 0; 0 0 1]  Quaternion=[1 0 0 0]  TranslationMethod=StandardAxis  TranslationCartesianOffset=[0 0 0]  TranslationCartesianOffsetUnits=m  TranslationStandardAxis=-Z  TranslationStandardOffset=len_shaft/4*rhs_shaft  TranslationStandardOffsetUnits=m  TranslationROffset=0  TranslationROffsetUnits=m  TranslationThetaOffset=0  TranslationThetaOffsetUnits=deg  TranslationZOffset=0  TranslationZOffsetUnits=m
  B : PMIOPort  Side=Left
  F : PMIOPort  Port=2  Side=Right
  meas : Outport  VectorParamsAs1DForOutWhenUnconnected=off
  wires:
  Bus Creator/1 -> meas/1
  PS-Simulink Converter/1 -> Bus Creator/2  "q"
  PS-Simulink Converter1/1 -> Bus Creator/1  "w"
  connections:
  PS-Simulink Converter1/LConn1 -- Revolute Flex/RConn3
  PS-Simulink Converter/LConn1 -- Revolute Flex/RConn2
  Transform SegF Ctr/LConn1 -- Revolute Flex/RConn1
  Transform SegF Ctr/RConn1 -- Shaft SegF/RConn1 -- Transform End/LConn1
  Transform SegB Ctr/RConn1 -- Shaft SegB/RConn1 -- Transform Ctr/LConn1
  Revolute Flex/LConn1 -- Transform Ctr/RConn1
  Transform SegB Ctr/LConn1 -- B/RConn1
  F/RConn1 -- Transform End/RConn1

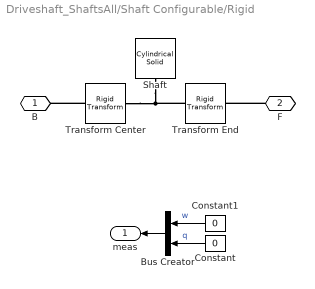
== system Driveshaft_ShaftsAll/Shaft Configurable/Rigid ==
  Bus Creator : BusCreator  Inputs=2
  Constant : Constant  Value=0
  Constant1 : Constant  Value=0
  Shaft : sm_lib/Body Elements/Cylindrical Solid  CylinderRadius=rad_shaft  CylinderRadiusUnits=m  CylinderLength=len_shaft  CylinderLengthUnits=m  ExportEntireGeometry=off  InertiaType=CalculateFromGeometry  BasedOnType=Mass  Density=1000  DensityUnits=kg/m^3  Mass=shaft_m  MassUnits=kg  CenterOfMass=[0 0 0]  CenterOfMassUnits=m  MomentsOfInertia=[1 1 1]  MomentsOfInertiaUnits=kg*m^2  ProductsOfInertia=[0 0 0]  ProductsOfInertiaUnits=kg*m^2  GraphicType=FromGeometry  MarkerShape=Sphere  MarkerSize=10  GraphicVisPropType=SimpleVisualProperties  GraphicDiffuseColor=clr_shaft  GraphicOpacity=opc_shaft  GraphicSpecularColor=[0.5 0.5 0.5 1.0]  GraphicAmbientColor=[0.15 0.15 0.15 1.0]  GraphicEmissiveColor=[0.0 0.0 0.0 1.0]  GraphicShininess=75  DoExposeReferenceFrame=on  SerializedFrames=<Frames/>
  Transform Center : sm_lib/Frames and Transforms/Rigid Transform  RotationMethod=None  FollAlignAxisA=+X  BaseAlignAxisA=+Y  FollAlignAxisB=+Y  BaseAlignAxisB=+Z  RotationStandardAxis=+Y  RotationAngle=0  RotationAngleUnits=deg  RotationArbitraryAxis=[0 0 1]  RotationSequenceAxes=FollowerAxes  RotationSequence=XYX  RotationSequenceAngles=[0 0 0]  RotationSequenceAnglesUnits=deg  RotationMatrix=[1 0 0; 0 1 0; 0 0 1]  Quaternion=[1 0 0 0]  TranslationMethod=StandardAxis  TranslationCartesianOffset=[0 0 0]  TranslationCartesianOffsetUnits=m  TranslationStandardAxis=-Z  TranslationStandardOffset=len_shaft/2*rhs_shaft  TranslationStandardOffsetUnits=m  TranslationROffset=0  TranslationROffsetUnits=m  TranslationThetaOffset=0  TranslationThetaOffsetUnits=deg  TranslationZOffset=0  TranslationZOffsetUnits=m
  Transform End : sm_lib/Frames and Transforms/Rigid Transform  RotationMethod=None  FollAlignAxisA=+X  BaseAlignAxisA=+Y  FollAlignAxisB=+Y  BaseAlignAxisB=+Z  RotationStandardAxis=+Y  RotationAngle=0  RotationAngleUnits=deg  RotationArbitraryAxis=[0 0 1]  RotationSequenceAxes=FollowerAxes  RotationSequence=XYX  RotationSequenceAngles=[0 0 0]  RotationSequenceAnglesUnits=deg  RotationMatrix=[1 0 0; 0 1 0; 0 0 1]  Quaternion=[1 0 0 0]  TranslationMethod=StandardAxis  TranslationCartesianOffset=[0 0 0]  TranslationCartesianOffsetUnits=m  TranslationStandardAxis=-Z  TranslationStandardOffset=len_shaft/2*rhs_shaft  TranslationStandardOffsetUnits=m  TranslationROffset=0  TranslationROffsetUnits=m  TranslationThetaOffset=0  TranslationThetaOffsetUnits=deg  TranslationZOffset=0  TranslationZOffsetUnits=m
  B : PMIOPort  Side=Left
  F : PMIOPort  Port=2  Side=Right
  meas : Outport  VectorParamsAs1DForOutWhenUnconnected=off
  wires:
  Bus Creator/1 -> meas/1
  Constant/1 -> Bus Creator/2  "q"
  Constant1/1 -> Bus Creator/1  "w"
  connections:
  Transform End/LConn1 -- Transform Center/RConn1 -- Shaft/RConn1
  Transform Center/LConn1 -- B/RConn1
  F/RConn1 -- Transform End/RConn1

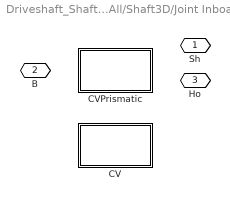
== system Driveshaft_ShaftsAll/Shaft3D/Joint Inboard ==
  CV : Subsystem  VariantControl=CV
  CVPrismatic : Subsystem  VariantControl=CVPrismatic
  " Sh" : PMIOPort  Side=Right
  " B" : PMIOPort  Port=2  Side=Left
  " Ho" : PMIOPort  Port=3  Side=Right

== system Driveshaft_ShaftsAll/Shaft3D/Joint Outboard ==
  CV : Subsystem  VariantControl=CV
  CVPrismatic : Subsystem  VariantControl=CVPrismatic
  " B" : PMIOPort  Side=Left
  " F" : PMIOPort  Port=2  Side=Right

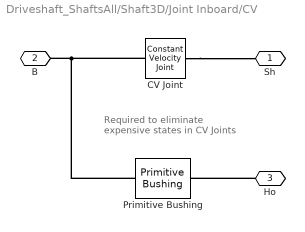
== system Driveshaft_ShaftsAll/Shaft3D/Joint Inboard/CV ==
  note: Required to eliminate
      | expensive states
      | in CV Joints
  CV Joint : sm_lib/Joints/Constant Velocity Joint  JointMode=Normal  CompositeWrenchDir=FollowerOnBase  CompositeWrenchFrame=BaseFrame  SenseConstraintForce=off  SenseConstraintTorque=off  SenseTotalForce=off  SenseTotalTorque=off  InternalState=Quaternion  PositionTargetSpecify=off  PositionTargetPriority=High  PositionTargetSpecificationMethod=BendAngleOnly  PositionTargetBendAngleValue=0.0  PositionTargetBendAngleValueUnits=deg  PositionTargetAzimuthValue=0.0  PositionTargetAzimuthValueUnits=deg  VelocityTargetSpecify=off  VelocityTargetPriority=High  VelocityTargetSpecificationMethod=BendAngleOnly  VelocityTargetBendAngleValue=0.0  VelocityTargetBendAngleValueUnits=deg/s  VelocityTargetAzimuthValue=0.0  VelocityTargetAzimuthValueUnits=deg/s  SenseBendAnglePosition=off  SenseBendAngleVelocity=off  SenseBendAngleAcceleration=off  SenseAzimuthPosition=off  SenseAzimuthVelocity=off  SenseAzimuthAcceleration=off
  Primitive Bushing : sm_car_lib/Utilities/Primitive Bushing  SystemSampleTime=-1  VariantActivationTime=update diagram  EmptyChoice=off  PassThrough=off  PassThroughVariantControl=(default)  EmptyChoiceVariantControl=(default)  AllowFlexibleInterface=on  Latency=0  AutoFrameSizeCalculation=off
  Sh : PMIOPort  Side=Right
  B : PMIOPort  Port=2  Side=Left
  Ho : PMIOPort  Port=3  Side=Right
  connections:
  Ho/RConn1 -- Primitive Bushing/LConn1
  CV Joint/LConn1 -- B/RConn1 -- Primitive Bushing/RConn1
  CV Joint/RConn1 -- Sh/RConn1

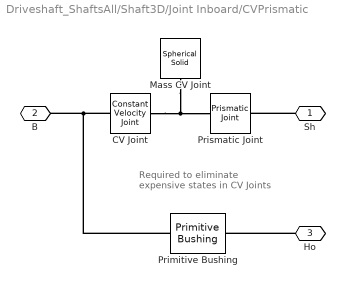
== system Driveshaft_ShaftsAll/Shaft3D/Joint Inboard/CVPrismatic ==
  note: Required to eliminate
      | expensive states
      | in CV Joints
  CV Joint : sm_lib/Joints/Constant Velocity Joint  JointMode=Normal  CompositeWrenchDir=FollowerOnBase  CompositeWrenchFrame=BaseFrame  SenseConstraintForce=off  SenseConstraintTorque=off  SenseTotalForce=off  SenseTotalTorque=off  InternalState=Quaternion  PositionTargetSpecify=off  PositionTargetPriority=High  PositionTargetSpecificationMethod=BendAngleOnly  PositionTargetBendAngleValue=0.0  PositionTargetBendAngleValueUnits=deg  PositionTargetAzimuthValue=0.0  PositionTargetAzimuthValueUnits=deg  VelocityTargetSpecify=off  VelocityTargetPriority=High  VelocityTargetSpecificationMethod=BendAngleOnly  VelocityTargetBendAngleValue=0.0  VelocityTargetBendAngleValueUnits=deg/s  VelocityTargetAzimuthValue=0.0  VelocityTargetAzimuthValueUnits=deg/s  SenseBendAnglePosition=off  SenseBendAngleVelocity=off  SenseBendAngleAcceleration=off  SenseAzimuthPosition=off  SenseAzimuthVelocity=off  SenseAzimuthAcceleration=off
  Mass CV Joint : sm_lib/Body Elements/Spherical Solid  SphereRadius=5e-3  SphereRadiusUnits=m  ExportEntireGeometry=off  InertiaType=CalculateFromGeometry  BasedOnType=Density  Density=1000  DensityUnits=kg/m^3  Mass=1  MassUnits=kg  CenterOfMass=[0 0 0]  CenterOfMassUnits=m  MomentsOfInertia=[1 1 1]  MomentsOfInertiaUnits=kg*m^2  ProductsOfInertia=[0 0 0]  ProductsOfInertiaUnits=kg*m^2  GraphicType=FromGeometry  MarkerShape=Sphere  MarkerSize=10  GraphicVisPropType=SimpleVisualProperties  GraphicDiffuseColor=[0.5 0.5 0.5]  GraphicOpacity=1  GraphicSpecularColor=[0.5 0.5 0.5 1.0]  GraphicAmbientColor=[0.15 0.15 0.15 1.0]  GraphicEmissiveColor=[0.0 0.0 0.0 1.0]  GraphicShininess=75  DoExposeReferenceFrame=on  SerializedFrames=<Frames/>
  Primitive Bushing : sm_car_lib/Utilities/Primitive Bushing  SystemSampleTime=-1  VariantActivationTime=update diagram  EmptyChoice=off  PassThrough=off  PassThroughVariantControl=(default)  EmptyChoiceVariantControl=(default)  AllowFlexibleInterface=on  Latency=0  AutoFrameSizeCalculation=off
  Prismatic Joint : sm_lib/Joints/Prismatic Joint  JointMode=Normal  CompositeWrenchDir=FollowerOnBase  CompositeWrenchFrame=BaseFrame  SenseConstraintForce=off  SenseConstraintTorque=off  SenseTotalForce=off  SenseTotalTorque=off  PositionTargetSpecify=off  PositionTargetPriority=High  PositionTargetValue=0  PositionTargetValueUnits=m  VelocityTargetSpecify=off  VelocityTargetPriority=High  VelocityTargetValue=0  VelocityTargetValueUnits=m/s  EquilibriumPosition=0  EquilibriumPositionUnits=m  SpringStiffness=0  SpringStiffnessUnits=N/m  DampingCoefficient=0  DampingCoefficientUnits=N/(m/s)  LowerLimitSpecify=off  LowerLimitBound=-1  LowerLimitBoundUnits=m  LowerLimitStiffness=1e6  LowerLimitStiffnessUnits=N/m  LowerLimitDamping=1e3  LowerLimitDampingUnits=N/(m/s)  LowerLimitTransitionRegionWidth=1e-4  LowerLimitTransitionRegionWidthUnits=m  UpperLimitSpecify=off  UpperLimitBound=1  UpperLimitBoundUnits=m  UpperLimitStiffness=1e6  UpperLimitStiffnessUnits=N/m  UpperLimitDamping=1e3  UpperLimitDampingUnits=N/(m/s)  UpperLimitTransitionRegionWidth=1e-4  UpperLimitTransitionRegionWidthUnits=m  TorqueActuationMode=NoTorque  MotionActuationMode=ComputedMotion  SensePosition=off  SenseVelocity=off  SenseAcceleration=off  SenseTorqueForce=off  SenseLowerLimitTorqueForce=off  SenseUpperLimitTorqueForce=off
  Sh : PMIOPort  Side=Right
  B : PMIOPort  Port=2  Side=Left
  Ho : PMIOPort  Port=3  Side=Right
  connections:
  Sh/RConn1 -- Prismatic Joint/RConn1
  CV Joint/RConn1 -- Prismatic Joint/LConn1 -- Mass CV Joint/RConn1
  CV Joint/LConn1 -- Primitive Bushing/RConn1 -- B/RConn1
  Ho/RConn1 -- Primitive Bushing/LConn1

== system Driveshaft_ShaftsAll/Shaft3D/Joint Outboard/CV ==
  CV Joint : sm_lib/Joints/Constant Velocity Joint  JointMode=Normal  CompositeWrenchDir=FollowerOnBase  CompositeWrenchFrame=BaseFrame  SenseConstraintForce=off  SenseConstraintTorque=off  SenseTotalForce=off  SenseTotalTorque=off  InternalState=Quaternion  PositionTargetSpecify=off  PositionTargetPriority=High  PositionTargetSpecificationMethod=BendAngleOnly  PositionTargetBendAngleValue=0.0  PositionTargetBendAngleValueUnits=deg  PositionTargetAzimuthValue=0.0  PositionTargetAzimuthValueUnits=deg  VelocityTargetSpecify=off  VelocityTargetPriority=High  VelocityTargetSpecificationMethod=BendAngleOnly  VelocityTargetBendAngleValue=0.0  VelocityTargetBendAngleValueUnits=deg/s  VelocityTargetAzimuthValue=0.0  VelocityTargetAzimuthValueUnits=deg/s  SenseBendAnglePosition=off  SenseBendAngleVelocity=off  SenseBendAngleAcceleration=off  SenseAzimuthPosition=off  SenseAzimuthVelocity=off  SenseAzimuthAcceleration=off
  B : PMIOPort  Side=Left
  F : PMIOPort  Port=2  Side=Right
  connections:
  CV Joint/LConn1 -- B/RConn1
  F/RConn1 -- CV Joint/RConn1

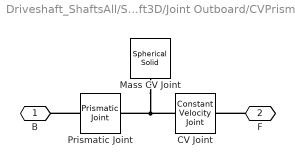
== system Driveshaft_ShaftsAll/Shaft3D/Joint Outboard/CVPrismatic ==
  CV Joint : sm_lib/Joints/Constant Velocity Joint  JointMode=Normal  CompositeWrenchDir=FollowerOnBase  CompositeWrenchFrame=BaseFrame  SenseConstraintForce=off  SenseConstraintTorque=off  SenseTotalForce=off  SenseTotalTorque=off  InternalState=Quaternion  PositionTargetSpecify=off  PositionTargetPriority=High  PositionTargetSpecificationMethod=BendAngleOnly  PositionTargetBendAngleValue=0.0  PositionTargetBendAngleValueUnits=deg  PositionTargetAzimuthValue=0.0  PositionTargetAzimuthValueUnits=deg  VelocityTargetSpecify=off  VelocityTargetPriority=High  VelocityTargetSpecificationMethod=BendAngleOnly  VelocityTargetBendAngleValue=0.0  VelocityTargetBendAngleValueUnits=deg/s  VelocityTargetAzimuthValue=0.0  VelocityTargetAzimuthValueUnits=deg/s  SenseBendAnglePosition=off  SenseBendAngleVelocity=off  SenseBendAngleAcceleration=off  SenseAzimuthPosition=off  SenseAzimuthVelocity=off  SenseAzimuthAcceleration=off
  Mass CV Joint : sm_lib/Body Elements/Spherical Solid  SphereRadius=5e-3  SphereRadiusUnits=m  ExportEntireGeometry=off  InertiaType=CalculateFromGeometry  BasedOnType=Density  Density=1*1000  DensityUnits=kg/m^3  Mass=1  MassUnits=kg  CenterOfMass=[0 0 0]  CenterOfMassUnits=m  MomentsOfInertia=[1 1 1]  MomentsOfInertiaUnits=kg*m^2  ProductsOfInertia=[0 0 0]  ProductsOfInertiaUnits=kg*m^2  GraphicType=FromGeometry  MarkerShape=Sphere  MarkerSize=10  GraphicVisPropType=SimpleVisualProperties  GraphicDiffuseColor=[0.5 0.5 0.5]  GraphicOpacity=1  GraphicSpecularColor=[0.5 0.5 0.5 1.0]  GraphicAmbientColor=[0.15 0.15 0.15 1.0]  GraphicEmissiveColor=[0.0 0.0 0.0 1.0]  GraphicShininess=75  DoExposeReferenceFrame=on  SerializedFrames=<Frames/>
  Prismatic Joint : sm_lib/Joints/Prismatic Joint  JointMode=Normal  CompositeWrenchDir=FollowerOnBase  CompositeWrenchFrame=BaseFrame  SenseConstraintForce=off  SenseConstraintTorque=off  SenseTotalForce=off  SenseTotalTorque=off  PositionTargetSpecify=off  PositionTargetPriority=High  PositionTargetValue=0  PositionTargetValueUnits=m  VelocityTargetSpecify=off  VelocityTargetPriority=High  VelocityTargetValue=0  VelocityTargetValueUnits=m/s  EquilibriumPosition=0  EquilibriumPositionUnits=m  SpringStiffness=0  SpringStiffnessUnits=N/m  DampingCoefficient=0  DampingCoefficientUnits=N/(m/s)  LowerLimitSpecify=off  LowerLimitBound=-1  LowerLimitBoundUnits=m  LowerLimitStiffness=1e6  LowerLimitStiffnessUnits=N/m  LowerLimitDamping=1e3  LowerLimitDampingUnits=N/(m/s)  LowerLimitTransitionRegionWidth=1e-4  LowerLimitTransitionRegionWidthUnits=m  UpperLimitSpecify=off  UpperLimitBound=1  UpperLimitBoundUnits=m  UpperLimitStiffness=1e6  UpperLimitStiffnessUnits=N/m  UpperLimitDamping=1e3  UpperLimitDampingUnits=N/(m/s)  UpperLimitTransitionRegionWidth=1e-4  UpperLimitTransitionRegionWidthUnits=m  TorqueActuationMode=NoTorque  MotionActuationMode=ComputedMotion  SensePosition=off  SenseVelocity=off  SenseAcceleration=off  SenseTorqueForce=off  SenseLowerLimitTorqueForce=off  SenseUpperLimitTorqueForce=off
  B : PMIOPort  Side=Left
  F : PMIOPort  Port=2  Side=Right
  connections:
  Prismatic Joint/LConn1 -- B/RConn1
  F/RConn1 -- CV Joint/RConn1
  Mass CV Joint/RConn1 -- CV Joint/LConn1 -- Prismatic Joint/RConn1
